simulink model "rocket_environment"  (R2022a)
settings: Solver=FixedStepAuto  StartTime=simtime(1)  StopTime=simtime(end)  FixedStep=dt  RelTol=1e-3
values from neighbouring files (symbols this model uses):
  dt = 1 / 100    (= 0.01)    [simulink_pre.m]
  I_T = openrocket.I    [simulink_pre.m]
  random_torque_rms = 1    [simulink_pre.m]
  s = size(dat)    [simulink_post.m]
  x_0 = openrocket.x.Data(1,:)    [simulink_pre.m]
undefined symbols (not defined in the file or in its folder): base, Discrete, filters, rotating_xy, rotating_xyz, Time
libraries: sm_lib x8, nesl_utility x7, sharedTrackingLibrary x3, eeGeneralControl x1, simulink x1, ctrlSharedLib x1
settings Model: Creator=yevge  LastModifiedBy=yevge
settings DiagnosticsConfigSet: SimMechanicsCrossSectionNullEdge=error  SimMechanicsUnconnectedFramePorts=none  SimMechanicsConflictingReferenceFrames=error  SimMechanicsUnsatisfiedHighPriorityTargets=error

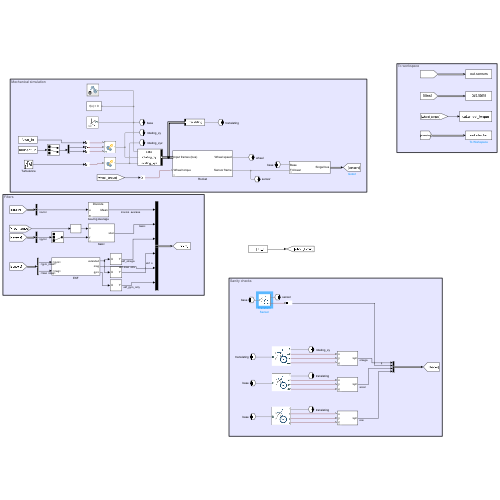
[thumbnail: Simulink's stored preview of the top-level diagram]
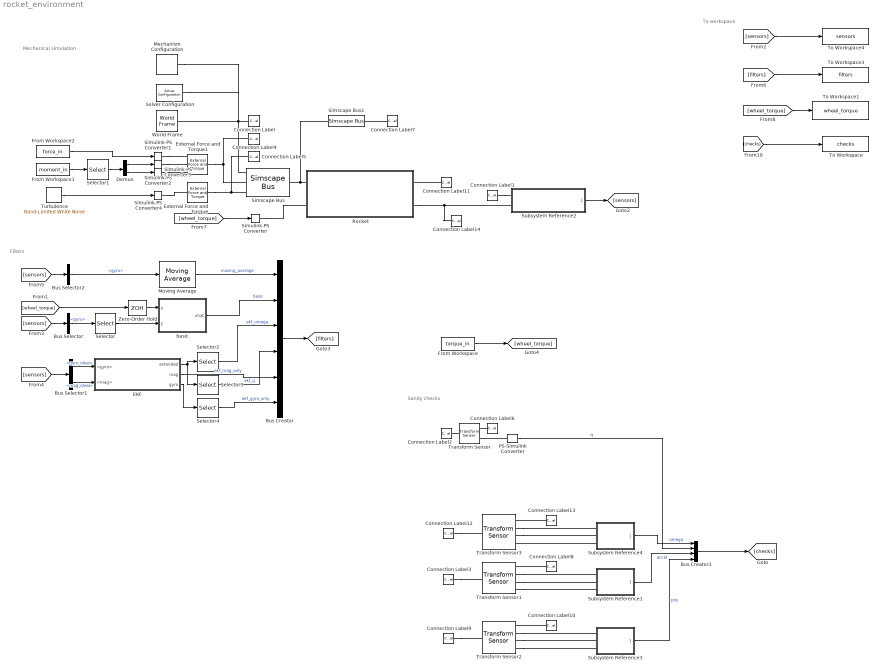
== system rocket_environment ==
  note: To workspace
  note: Sanity checks
  note: Filters
  note: Mechanical simulation
  Bus Creator : BusCreator  Inputs=6
  Bus Creator1 : BusCreator  Inputs=4
  Bus Selector : BusSelector  OutputSignals=gyro
  Bus Selector1 : BusSelector  OutputSignals=gyro_ideal,mag_ideal
  Bus Selector2 : BusSelector  OutputSignals=gyro
  Connection Label{,1..3,9} (5 alike) : ConnectionLabel  Label=base
  Connection Label{7..8,10,12} (4 alike) : ConnectionLabel  Label=translating
  Connection Label11 : ConnectionLabel  Label=wheel
  Connection Label13 : ConnectionLabel  Label=rotating_xy
  Connection Label14 : ConnectionLabel  Label=sensor
  Connection Label4 : ConnectionLabel  Label=rotating_xy
  Connection Label5 : ConnectionLabel  Label=rotating_xyz
  Connection Label6 : ConnectionLabel  Label=sensor
  Demux : Demux  Outputs=2
  EKF : Subsystem  mask{filter_params=filters.ekf}
      mask prompts: filter_params "Filter parameter structure"
  External Force and Torque : sm_lib/Forces and Torques/External Force and Torque  ForceResolutionFrame=World  EnableForceX=off  EnableForceY=off  EnableForceZ=off  EnableForce=off  TorqueResolutionFrame=AttachedFrame  EnableTorqueX=off  EnableTorqueY=off  EnableTorqueZ=on  EnableTorque=off
  External Force and Torque1 : sm_lib/Forces and Torques/External Force and Torque  ForceResolutionFrame=World  EnableForceX=off  EnableForceY=off  EnableForceZ=off  EnableForce=on  TorqueResolutionFrame=AttachedFrame  EnableTorqueX=on  EnableTorqueY=on  EnableTorqueZ=off  EnableTorque=off
  From Workspace : FromWorkspace  VariableName=torque_in
  From Workspace1 : FromWorkspace  VariableName=moment_in  OutputAfterFinalValue=Setting to zero
  From Workspace2 : FromWorkspace  VariableName=force_in  OutputAfterFinalValue=Setting to zero
  Mechanism Configuration : sm_lib/Utilities/Mechanism Configuration  UniformGravity=None  GravityVector=[0 0 -9.80665]  GravityUnits=m/s^2  LinearizationDelta=0.001  JointModeTransitionNonlinearIterations=2
  Moving Average : eeGeneralControl/Moving Average  VariantControl=Variant1  LabelModeActiveChoice=Discrete  f=[10 10 10]  x0=0  BufferSize=8192  Ts=-1
      settings: SourceProductBaseCode=PS
  PS-Simulink Converter : nesl_utility/PS-Simulink Converter  PhysicalDomain=network_engine_domain  SubClassName=ps_output  LeftPortType=input  RightPortType=output  PseudoPeriodic=off  Frequencies=[]  VectorFormat=inherit  Unit=inherit  AffineConversion=off
      settings: SourceProductBaseCode=SS,PW,VE
  Rocket : Subsystem  ReferencedSubsystem=rocket  M_T=M_T  Iz_T=I_T(3)  Ix_T=I_T(2)  L_R=322  CG=161  M_W=0  I_W=I_W  tilt=0  X_W=87.6  X0=x_0  V0=v_0  THETA0=theta_0  OMEGA0=omega_0
  Selector : Selector  InputPortWidth=3  IndexOptions=Index vector (dialog)  Indices=3  OutputSizes=1
  Selector1 : Selector  InputPortWidth=3  IndexOptions=Index vector (dialog)  Indices=[1 2]  OutputSizes=1
  Selector2 : Selector  InputPortWidth=7  IndexOptions=Index vector (dialog)  Indices=1:3  OutputSizes=1
  Selector3 : Selector  InputPortWidth=7  IndexOptions=Index vector (dialog)  Indices=4:7  OutputSizes=1
  Selector4 : Selector  InputPortWidth=7  IndexOptions=Index vector (dialog)  Indices=4:7  OutputSizes=1
  Simscape Bus : SimscapeBus  HierarchyStrings=base;rotating_xy;rotating_xyz
  Simscape Bus1 : SimscapeBus  HierarchyStrings=translating
  Simulink-PS Converter{,2..4} (4 alike) : nesl_utility/Simulink-PS Converter  PhysicalDomain=network_engine_domain  SubClassName=ps_input  LeftPortType=input  RightPortType=output  PseudoPeriodic=off  Frequencies=[]  NoiseDistribution=none  NoiseParameters=[]  Unit=N*m  AffineConversion=on  FilteringAndDerivatives=provide  SimscapeFilterOrder=1  InputFilterTimeConstant=0.001  UdotUserProvided=0
      settings: SourceProductBaseCode=SS,PW,VE
  Simulink-PS Converter1 : nesl_utility/Simulink-PS Converter  PhysicalDomain=network_engine_domain  SubClassName=ps_input  LeftPortType=input  RightPortType=output  PseudoPeriodic=off  Frequencies=[]  NoiseDistribution=none  NoiseParameters=[]  Unit=N  AffineConversion=on  FilteringAndDerivatives=provide  SimscapeFilterOrder=1  InputFilterTimeConstant=0.001  UdotUserProvided=0
      settings: SourceProductBaseCode=SS,PW,VE
  Solver Configuration : nesl_utility/Solver Configuration  PhysicalDomain=network_engine_domain  SubClassName=solver  LeftPortType=input  RightPortType=generic  Tones=[]  Harmonics=[]  SimulateNoise=off  Profile=off  UseLocalSampling=off  EnableSwitchedLinearOptims=on  FrequencyDomain=off  UseCCode=off  RelTol=0.001  AbsTol=0.001  MinStep=1e-09  ToWorkspace=off  RevertToSquareIcSolve=off  NumHomotopyIterations=100  PhasorMode=off  PhasorModeNumHarmonics=1  IndexReductionMethod=DerivativeReplacement  DoDC=off  ResidualTolerance=1e-09  UseLocalSolver=off  LocalSolverChoice=NE_BACKWARD_EULER_ADVANCER  LocalSolverSampleTime=0.001  DoFixedCost=off  MaxNonlinIter=3  MaxModeIter=2  ComputeImpulses=off  ImpulseIterations=2  LinearAlgebra=auto  LinearAlgebraNumThread=0  EquationFormulation=NE_TIME_EF  DelaysMemoryBudget=1024  AutomaticFiltering=on  FilteringTimeConstant=0.001  PartitionStorageMethod=AS_NEEDED  PartitionMemoryBudget=1024  PartitionMethod=ROBUST
      settings: SourceProductBaseCode=SS,PW,VE
  Subsystem Reference1 : Subsystem  ReferencedSubsystem=PS_Simulink_3x  Unit=m/s^2
  Subsystem Reference2 : Subsystem  ReferencedSubsystem=sensors  rg=gyro_rms  rtg=gyro_drift_rms  ra=accel_rms  rm=mag_rms  B0=mag_field_0  dt=dt
  Subsystem Reference3 : Subsystem  ReferencedSubsystem=PS_Simulink_3x  Unit=m
  Subsystem Reference4 : Subsystem  ReferencedSubsystem=PS_Simulink_3x  Unit=rad/s
  To Workspace : ToWorkspace  VariableName=checks  SaveFormat=Timeseries  SampleTime=-1
  To Workspace1 : ToWorkspace  VariableName=wheel_torque  SaveFormat=Timeseries  SampleTime=-1
  To Workspace3 : ToWorkspace  VariableName=filters  SaveFormat=Timeseries  SampleTime=-1
  To Workspace4 : ToWorkspace  VariableName=sensors  SaveFormat=Timeseries  SampleTime=-1
  Transform Sensor : sm_lib/Frames and Transforms/Transform Sensor  MeasurementFrame=Follower  SenseAngle=off  SenseAxis=off  SenseAngle1=off  SenseAngle2=off  SenseAngle3=off  SenseQ=on  SenseR=off  SenseOmegaX=off  SenseOmegaY=off  SenseOmegaZ=off  SenseOmega1=off  SenseOmega2=off  SenseOmega3=off  SenseQDot=off  SenseRDot=off  SenseAlphaX=off  SenseAlphaY=off  SenseAlphaZ=off  SenseAlpha1=off  SenseAlpha2=off  SenseAlpha3=off  SenseQDDot=off  SenseRDDot=off  SenseX=off  SenseY=off  SenseZ=off  SenseRad=off  SenseAzim=off  SenseDist=off  SenseInc=off  SenseXDot=off  SenseYDot=off  SenseZDot=off  SenseRadDot=off  SenseAzimDot=off  SenseDistDot=off  SenseIncDot=off  SenseXDDot=off  SenseYDDot=off  SenseZDDot=off  SenseRadDDot=off  SenseAzimDDot=off  SenseDistDDot=off  SenseIncDDot=off
  Transform Sensor1 : sm_lib/Frames and Transforms/Transform Sensor  MeasurementFrame=Base  SenseAngle=off  SenseAxis=off  SenseAngle1=off  SenseAngle2=off  SenseAngle3=off  SenseQ=off  SenseR=off  SenseOmegaX=off  SenseOmegaY=off  SenseOmegaZ=off  SenseOmega1=off  SenseOmega2=off  SenseOmega3=off  SenseQDot=off  SenseRDot=off  SenseAlphaX=off  SenseAlphaY=off  SenseAlphaZ=off  SenseAlpha1=off  SenseAlpha2=off  SenseAlpha3=off  SenseQDDot=off  SenseRDDot=off  SenseX=off  SenseY=off  SenseZ=off  SenseRad=off  SenseAzim=off  SenseDist=off  SenseInc=off  SenseXDot=off  SenseYDot=off  SenseZDot=off  SenseRadDot=off  SenseAzimDot=off  SenseDistDot=off  SenseIncDot=off  SenseXDDot=on  SenseYDDot=on  SenseZDDot=on  SenseRadDDot=off  SenseAzimDDot=off  SenseDistDDot=off  SenseIncDDot=off
  Transform Sensor2 : sm_lib/Frames and Transforms/Transform Sensor  MeasurementFrame=Base  SenseAngle=off  SenseAxis=off  SenseAngle1=off  SenseAngle2=off  SenseAngle3=off  SenseQ=off  SenseR=off  SenseOmegaX=off  SenseOmegaY=off  SenseOmegaZ=off  SenseOmega1=off  SenseOmega2=off  SenseOmega3=off  SenseQDot=off  SenseRDot=off  SenseAlphaX=off  SenseAlphaY=off  SenseAlphaZ=off  SenseAlpha1=off  SenseAlpha2=off  SenseAlpha3=off  SenseQDDot=off  SenseRDDot=off  SenseX=on  SenseY=on  SenseZ=on  SenseRad=off  SenseAzim=off  SenseDist=off  SenseInc=off  SenseXDot=off  SenseYDot=off  SenseZDot=off  SenseRadDot=off  SenseAzimDot=off  SenseDistDot=off  SenseIncDot=off  SenseXDDot=off  SenseYDDot=off  SenseZDDot=off  SenseRadDDot=off  SenseAzimDDot=off  SenseDistDDot=off  SenseIncDDot=off
  Transform Sensor3 : sm_lib/Frames and Transforms/Transform Sensor  MeasurementFrame=Follower  SenseAngle=off  SenseAxis=off  SenseAngle1=off  SenseAngle2=off  SenseAngle3=off  SenseQ=off  SenseR=off  SenseOmegaX=on  SenseOmegaY=on  SenseOmegaZ=on  SenseOmega1=off  SenseOmega2=off  SenseOmega3=off  SenseQDot=off  SenseRDot=off  SenseAlphaX=off  SenseAlphaY=off  SenseAlphaZ=off  SenseAlpha1=off  SenseAlpha2=off  SenseAlpha3=off  SenseQDDot=off  SenseRDDot=off  SenseX=off  SenseY=off  SenseZ=off  SenseRad=off  SenseAzim=off  SenseDist=off  SenseInc=off  SenseXDot=off  SenseYDot=off  SenseZDot=off  SenseRadDot=off  SenseAzimDot=off  SenseDistDot=off  SenseIncDot=off  SenseXDDot=off  SenseYDDot=off  SenseZDDot=off  SenseRadDDot=off  SenseAzimDDot=off  SenseDistDDot=off  SenseIncDDot=off
  Turbulence : simulink/Sources/Band-Limited White Noise  Cov=random_torque_rms .^ 2 * dt  Ts=dt  seed=randi(10000,1)
  World Frame : sm_lib/Frames and Transforms/World Frame
  Zero-Order Hold : ZeroOrderHold  SampleTime=dt
  basic : Subsystem  mask{filter_params=filters.basic}
      mask prompts: filter_params "Filter parameter structure"
  wires:
  From Workspace2/1 -> Simulink-PS Converter1/1
  Turbulence/1 -> Simulink-PS Converter4/1
  Subsystem Reference2/1 -> [sensors]
  Bus Selector/1 -> Selector/1  "<gyro>"
  Selector1/1 -> Demux/1
  From Workspace1/1 -> Selector1/1
  Demux/1 -> Simulink-PS Converter2/1
  Demux/2 -> Simulink-PS Converter3/1
  [sensors] -> To Workspace4/1
  [sensors] -> Bus Selector/1
  Bus Creator/1 -> [filters]
  [filters] -> To Workspace3/1
  [wheel_torque] -> Simulink-PS Converter/1
  [wheel_torque] -> To Workspace1/1
  From Workspace/1 -> [wheel_torque]
  PS-Simulink Converter/1 -> Bus Creator1/2  "q"
  Bus Creator1/1 -> [checks]
  [checks] -> To Workspace/1
  [sensors] -> Bus Selector1/1
  Bus Selector1/1 -> EKF/1(<gyro>)  "<gyro_ideal>"
  Bus Selector1/2 -> EKF/2(<mag>)  "<mag_ideal>"
  Subsystem Reference1/1 -> Bus Creator1/3  "accel"
  Subsystem Reference3/1 -> Bus Creator1/4  "pos"
  [wheel_torque] -> Zero-Order Hold/1
  Selector/1 -> basic/2(y)
  basic/1(xhat) -> Bus Creator/2  "basic"
  EKF/1(extended) -> Selector3/1, Selector2/1
  Selector2/1 -> Bus Creator/3  "ekf_omega"
  Selector3/1 -> Bus Creator/4  "ekf_q"
  [sensors] -> Bus Selector2/1
  Bus Selector2/1 -> Moving Average/1  "<gyro>"
  Moving Average/1 -> Bus Creator/1  "moving_average"
  Subsystem Reference4/1 -> Bus Creator1/1  "omega"
  Zero-Order Hold/1 -> basic/1(u)
  EKF/2(mag) -> Bus Creator/5  "ekf_mag_only"
  EKF/3(gyro) -> Selector4/1
  Selector4/1 -> Bus Creator/6  "ekf_gyro_only"
  connections:
  Mechanism Configuration/RConn1 -- Solver Configuration/RConn1 -- Connection Label/LConn1 -- Simscape Bus/LConn1 -- World Frame/RConn1
  Simulink-PS Converter1/RConn1 -- External Force and Torque1/LConn1
  Simulink-PS Converter4/RConn1 -- External Force and Torque/LConn1
  Simulink-PS Converter3/RConn1 -- External Force and Torque1/LConn3
  Simulink-PS Converter2/RConn1 -- External Force and Torque1/LConn2
  Rocket/LConn1 -- Simscape Bus1/RConn1 -- Simscape Bus/RConn1
  External Force and Torque1/RConn1 -- Simscape Bus/LConn2 -- Connection Label4/LConn1
  External Force and Torque/RConn1 -- Connection Label5/LConn1 -- Simscape Bus/LConn3
  Simulink-PS Converter/RConn1 -- Rocket/LConn2
  Rocket/RConn2 -- Connection Label14/LConn1 -- Subsystem Reference2/LConn2
  Connection Label1/LConn1 -- Subsystem Reference2/LConn1
  PS-Simulink Converter/LConn1 -- Transform Sensor/RConn2
  Connection Label6/LConn1 -- Transform Sensor/RConn1
  Connection Label2/LConn1 -- Transform Sensor/LConn1
  Connection Label3/LConn1 -- Transform Sensor1/LConn1
  Connection Label7/LConn1 -- Simscape Bus1/LConn1
  Connection Label8/LConn1 -- Transform Sensor1/RConn1
  Transform Sensor1/RConn2 -- Subsystem Reference1/LConn1
  Transform Sensor1/RConn3 -- Subsystem Reference1/LConn2
  Transform Sensor1/RConn4 -- Subsystem Reference1/LConn3
  Transform Sensor2/RConn4 -- Subsystem Reference3/LConn3
  Transform Sensor2/RConn2 -- Subsystem Reference3/LConn1
  Transform Sensor2/RConn3 -- Subsystem Reference3/LConn2
  Connection Label10/LConn1 -- Transform Sensor2/RConn1
  Connection Label9/LConn1 -- Transform Sensor2/LConn1
  Connection Label11/LConn1 -- Rocket/RConn1
  Transform Sensor3/RConn2 -- Subsystem Reference4/LConn1
  Connection Label13/LConn1 -- Transform Sensor3/RConn1
  Subsystem Reference4/LConn3 -- Transform Sensor3/RConn4
  Transform Sensor3/RConn3 -- Subsystem Reference4/LConn2
  Connection Label12/LConn1 -- Transform Sensor3/LConn1

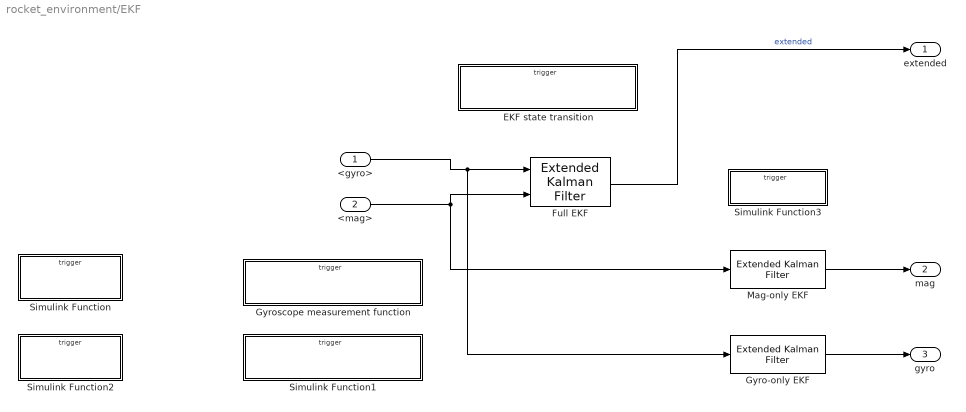
== system rocket_environment/EKF ==
  <gyro> : Inport
  <mag> : Inport  Port=2
  EKF state transition : Subsystem  TreatAsAtomicUnit=on
  Full EKF : sharedTrackingLibrary/Extended Kalman Filter  StateTransitionFcn=ekf_state_transition  HasStateTransitionJacobianFcn=off  HasAdditiveProcessNoise=Additive  ProcessNoise=filter_params.Q  HasTimeVaryingProcessNoise=off  HasStateTransitionFcnExtraArgument=0  InitialState=filter_params.X0  InitialStateCovariance=filter_params.Q0  MeasurementFcn1=gyro_update_sel  HasMeasurementJacobianFcn1=off  HasMeasurementEnablePort1=off  HasAdditiveMeasurementNoise1=Additive  MeasurementNoise1=filter_params.RG  HasTimeVaryingMeasurementNoise1=off  HasMeasurementFcnExtraArgument1=0  HasMeasurementWrapping1=off  MeasurementFcn2=mag_update_sel  HasMeasurementJacobianFcn2=off  HasMeasurementEnablePort2=off  HasAdditiveMeasurementNoise2=Additive  MeasurementNoise2=filter_params.RM  HasTimeVaryingMeasurementNoise2=off  HasMeasurementFcnExtraArgument2=0  HasMeasurementWrapping2=off  MeasurementFcn3=myMeasurementFcn  HasMeasurementJacobianFcn3=off  HasMeasurementEnablePort3=off  HasAdditiveMeasurementNoise3=Additive  MeasurementNoise3=1  HasTimeVaryingMeasurementNoise3=off  HasMeasurementFcnExtraArgument3=0  HasMeasurementWrapping3=off  MeasurementFcn4=myMeasurementFcn  HasMeasurementJacobianFcn4=off  HasMeasurementEnablePort4=off  HasAdditiveMeasurementNoise4=Additive  MeasurementNoise4=1  HasTimeVaryingMeasurementNoise4=off  HasMeasurementFcnExtraArgument4=0  HasMeasurementWrapping4=off  MeasurementFcn5=myMeasurementFcn  HasMeasurementJacobianFcn5=off  HasMeasurementEnablePort5=off  HasAdditiveMeasurementNoise5=Additive  MeasurementNoise5=1  HasTimeVaryingMeasurementNoise5=off  HasMeasurementFcnExtraArgument5=0  HasMeasurementWrapping5=off  EnableMultirate=off  StateTransitionFcnSampleTime=1  MeasurementFcn1SampleTime=1  MeasurementFcn2SampleTime=1  MeasurementFcn3SampleTime=1  MeasurementFcn4SampleTime=1  MeasurementFcn5SampleTime=1  UseCurrentEstimator=on  OutputStateCovariance=off  DataType=double  SampleTime=dt  NumberOfMeasurements=2
      settings: SourceProductBaseCode=TF,AE,PW,CT,DR,ID,LP,NV,AR,RO,RR,UV,VE
  Gyro-only EKF : sharedTrackingLibrary/Extended Kalman Filter  StateTransitionFcn=ekf_state_transition  HasStateTransitionJacobianFcn=off  HasAdditiveProcessNoise=Additive  ProcessNoise=eye(7) * 1e0  HasTimeVaryingProcessNoise=off  HasStateTransitionFcnExtraArgument=0  InitialState=filter_params.X0  InitialStateCovariance=eye(7) * 1e0  MeasurementFcn1=gyro_update_sel  HasMeasurementJacobianFcn1=off  HasMeasurementEnablePort1=off  HasAdditiveMeasurementNoise1=Additive  MeasurementNoise1=filter_params.RG * 1e-10  HasTimeVaryingMeasurementNoise1=off  HasMeasurementFcnExtraArgument1=0  HasMeasurementWrapping1=off  MeasurementFcn2=myMeasurementFcn  HasMeasurementJacobianFcn2=off  HasMeasurementEnablePort2=off  HasAdditiveMeasurementNoise2=Additive  MeasurementNoise2=1  HasTimeVaryingMeasurementNoise2=off  HasMeasurementFcnExtraArgument2=0  HasMeasurementWrapping2=off  MeasurementFcn3=myMeasurementFcn  HasMeasurementJacobianFcn3=off  HasMeasurementEnablePort3=off  HasAdditiveMeasurementNoise3=Additive  MeasurementNoise3=1  HasTimeVaryingMeasurementNoise3=off  HasMeasurementFcnExtraArgument3=0  HasMeasurementWrapping3=off  MeasurementFcn4=myMeasurementFcn  HasMeasurementJacobianFcn4=off  HasMeasurementEnablePort4=off  HasAdditiveMeasurementNoise4=Additive  MeasurementNoise4=1  HasTimeVaryingMeasurementNoise4=off  HasMeasurementFcnExtraArgument4=0  HasMeasurementWrapping4=off  MeasurementFcn5=myMeasurementFcn  HasMeasurementJacobianFcn5=off  HasMeasurementEnablePort5=off  HasAdditiveMeasurementNoise5=Additive  MeasurementNoise5=1  HasTimeVaryingMeasurementNoise5=off  HasMeasurementFcnExtraArgument5=0  HasMeasurementWrapping5=off  EnableMultirate=off  StateTransitionFcnSampleTime=1  MeasurementFcn1SampleTime=1  MeasurementFcn2SampleTime=1  MeasurementFcn3SampleTime=1  MeasurementFcn4SampleTime=1  MeasurementFcn5SampleTime=1  UseCurrentEstimator=on  OutputStateCovariance=off  DataType=double  SampleTime=dt  NumberOfMeasurements=1
      settings: SourceProductBaseCode=TF,AE,PW,CT,DR,ID,LP,NV,AR,RO,RR,UV,VE
  Gyroscope measurement function : Subsystem  TreatAsAtomicUnit=on
  Mag-only EKF : sharedTrackingLibrary/Extended Kalman Filter  StateTransitionFcn=state_identity  HasStateTransitionJacobianFcn=off  HasAdditiveProcessNoise=Additive  ProcessNoise=eye(4) * 1e0  HasTimeVaryingProcessNoise=off  HasStateTransitionFcnExtraArgument=0  InitialState=[-0.999; 0; -0.0436; 0]  InitialStateCovariance=eye(4) * 1e-2  MeasurementFcn1=mag_update  HasMeasurementJacobianFcn1=off  HasMeasurementEnablePort1=off  HasAdditiveMeasurementNoise1=Additive  MeasurementNoise1=filter_params.RM * 1e-10  HasTimeVaryingMeasurementNoise1=off  HasMeasurementFcnExtraArgument1=0  HasMeasurementWrapping1=off  MeasurementFcn2=myMeasurementFcn  HasMeasurementJacobianFcn2=off  HasMeasurementEnablePort2=off  HasAdditiveMeasurementNoise2=Additive  MeasurementNoise2=1  HasTimeVaryingMeasurementNoise2=off  HasMeasurementFcnExtraArgument2=0  HasMeasurementWrapping2=off  MeasurementFcn3=myMeasurementFcn  HasMeasurementJacobianFcn3=off  HasMeasurementEnablePort3=off  HasAdditiveMeasurementNoise3=Additive  MeasurementNoise3=1  HasTimeVaryingMeasurementNoise3=off  HasMeasurementFcnExtraArgument3=0  HasMeasurementWrapping3=off  MeasurementFcn4=myMeasurementFcn  HasMeasurementJacobianFcn4=off  HasMeasurementEnablePort4=off  HasAdditiveMeasurementNoise4=Additive  MeasurementNoise4=1  HasTimeVaryingMeasurementNoise4=off  HasMeasurementFcnExtraArgument4=0  HasMeasurementWrapping4=off  MeasurementFcn5=myMeasurementFcn  HasMeasurementJacobianFcn5=off  HasMeasurementEnablePort5=off  HasAdditiveMeasurementNoise5=Additive  MeasurementNoise5=1  HasTimeVaryingMeasurementNoise5=off  HasMeasurementFcnExtraArgument5=0  HasMeasurementWrapping5=off  EnableMultirate=off  StateTransitionFcnSampleTime=1  MeasurementFcn1SampleTime=1  MeasurementFcn2SampleTime=1  MeasurementFcn3SampleTime=1  MeasurementFcn4SampleTime=1  MeasurementFcn5SampleTime=1  UseCurrentEstimator=on  OutputStateCovariance=off  DataType=double  SampleTime=dt  NumberOfMeasurements=1
      settings: SourceProductBaseCode=TF,AE,PW,CT,DR,ID,LP,NV,AR,RO,RR,UV,VE
  Simulink Function : Subsystem  TreatAsAtomicUnit=on
  Simulink Function1 : Subsystem  TreatAsAtomicUnit=on
  Simulink Function2 : Subsystem  TreatAsAtomicUnit=on
  Simulink Function3 : Subsystem  TreatAsAtomicUnit=on
  extended : Outport
  mag : Outport  Port=2
  gyro : Outport  Port=3
  wires:
  Full EKF/1 -> extended/1  "extended"
  <gyro>/1 -> Gyro-only EKF/1, Full EKF/1
  <mag>/1 -> Full EKF/2, Mag-only EKF/1
  Mag-only EKF/1 -> mag/1
  Gyro-only EKF/1 -> gyro/1

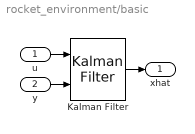
== system rocket_environment/basic ==
  u : Inport
  y : Inport  Port=2
  Kalman Filter : ctrlSharedLib/Kalman Filter  TimeDomain=Discrete-Time  UseCurrentEstimator=on  ModelSource=Individual A, B, C, D matrices  ModelSourceVariable=ss(0.95,1,1,0,1)  A=filter_params.A  B=filter_params.B  C=filter_params.C  D=filter_params.D  NumberOfStates=1  NumberOfInputs=1  NumberOfOutputs=1  InitialEstimateSource=Dialog  X0=filter_params.X0  P0=10  UseK=off  UseGH=off  NumberOfProcessNoiseInputs=1  G=1  TimeInvariantG=on  H=0  TimeInvariantH=on  Q=filter_params.Q  TimeInvariantQ=on  R=filter_params.R  TimeInvariantR=on  N=0  TimeInvariantN=on  AddInputPort=on  AddEnablePort=off  OutputEstimatedY=off  OutputP=off  Ts=dt
  xhat : Outport
  wires:
  Kalman Filter/1 -> xhat/1
  y/1 -> Kalman Filter/2
  u/1 -> Kalman Filter/1

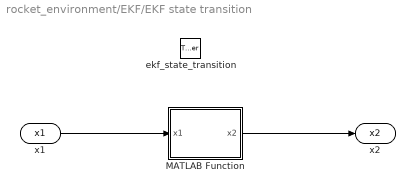
== system rocket_environment/EKF/EKF state transition ==
  ekf_state_transition : TriggerPort  TriggerType=function-call  IsSimulinkFunction=on  FunctionName=ekf_state_transition  FunctionVisibility=scoped  VariantControl=(inherit)
  MATLAB Function : MATLAB Function  TreatAsAtomicUnit=on
  x1 : ArgIn  DisableCoverage=on  PortDimensions=7  ArgumentName=x1
  x2 : ArgOut  DisableCoverage=on  PortDimensions=7  ArgumentName=x2
  wires:
  x1/1 -> MATLAB Function/1(x1)
  MATLAB Function/1(x2) -> x2/1

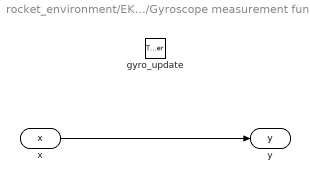
== system rocket_environment/EKF/Gyroscope measurement function ==
  gyro_update : TriggerPort  TriggerType=function-call  IsSimulinkFunction=on  FunctionName=gyro_update  FunctionVisibility=scoped  VariantControl=(inherit)
  x : ArgIn  DisableCoverage=on  PortDimensions=3  ArgumentName=x
  y : ArgOut  DisableCoverage=on  PortDimensions=3  ArgumentName=y
  wires:
  x/1 -> y/1

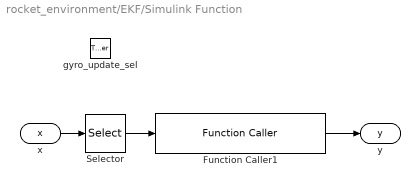
== system rocket_environment/EKF/Simulink Function ==
  gyro_update_sel : TriggerPort  TriggerType=function-call  IsSimulinkFunction=on  FunctionName=gyro_update_sel  FunctionVisibility=scoped  VariantControl=(inherit)
  Function Caller1 : FunctionCaller  FunctionPrototype=y = EKF.gyro_update(x)  InputArgumentSpecifications=<Enter example>  OutputArgumentSpecifications=<Enter example>
  Selector : Selector  InputPortWidth=7  IndexOptions=Index vector (dialog)  Indices=1:3  OutputSizes=1
  x : ArgIn  DisableCoverage=on  PortDimensions=7  ArgumentName=x
  y : ArgOut  DisableCoverage=on  PortDimensions=3  ArgumentName=y
  wires:
  x/1 -> Selector/1
  Selector/1 -> Function Caller1/1
  Function Caller1/1 -> y/1

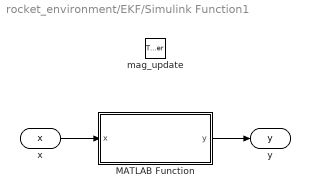
== system rocket_environment/EKF/Simulink Function1 ==
  mag_update : TriggerPort  TriggerType=function-call  IsSimulinkFunction=on  FunctionName=mag_update  FunctionVisibility=scoped  VariantControl=(inherit)
  MATLAB Function : MATLAB Function  TreatAsAtomicUnit=on
  x : ArgIn  DisableCoverage=on  PortDimensions=4  ArgumentName=x
  y : ArgOut  DisableCoverage=on  PortDimensions=3  ArgumentName=y
  wires:
  x/1 -> MATLAB Function/1(x)
  MATLAB Function/1(y) -> y/1

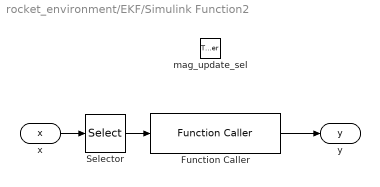
== system rocket_environment/EKF/Simulink Function2 ==
  mag_update_sel : TriggerPort  TriggerType=function-call  IsSimulinkFunction=on  FunctionName=mag_update_sel  FunctionVisibility=scoped  VariantControl=(inherit)
  Function Caller : FunctionCaller  FunctionPrototype=y = EKF.mag_update(x)  InputArgumentSpecifications=<Enter example>  OutputArgumentSpecifications=<Enter example>
  Selector : Selector  InputPortWidth=7  IndexOptions=Index vector (dialog)  Indices=4:7  OutputSizes=1
  x : ArgIn  DisableCoverage=on  PortDimensions=7  ArgumentName=x
  y : ArgOut  DisableCoverage=on  PortDimensions=3  ArgumentName=y
  wires:
  x/1 -> Selector/1
  Function Caller/1 -> y/1
  Selector/1 -> Function Caller/1

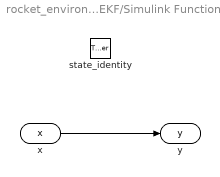
== system rocket_environment/EKF/Simulink Function3 ==
  state_identity : TriggerPort  TriggerType=function-call  IsSimulinkFunction=on  FunctionName=state_identity  FunctionVisibility=scoped  VariantControl=(inherit)
  x : ArgIn  DisableCoverage=on  PortDimensions=4  ArgumentName=x
  y : ArgOut  DisableCoverage=on  PortDimensions=4  ArgumentName=y
  wires:
  x/1 -> y/1

== matlab function rocket_environment/EKF/Simulink Function1/MATLAB Function ==
  data: x input; y output; B0 parameter
function y = mag_measurement(x, B0)
    y = rotateframe(quaternion(x'), B0);
end

== matlab function rocket_environment/EKF/EKF state transition/MATLAB Function ==
  data: x1 input; x2 output; dt parameter
function x2 = state(x1, dt)
    x1 = x1';
    q_1 = quaternion(x1(4:7)); % orientation quaternion

    q_omega = quaternion([0 x1(1:3)]); % rate quaternion
    

    q_rate = - 0.5 * q_1 * q_omega; % orientation time-derivative
    q_2 = q_1 + (dt * q_rate); % update

    
    x2 = [x1(1:3) compact(q_2)]';
end
